simulink model "HTdieukhiennhietdophong"  (R2017b)
settings: Solver=VariableStepAuto  StartTime=0.0  StopTime=200  RelTol=1e-3
libraries: simulink x2
settings Model: Creator=chemi  LastModifiedBy=chemi

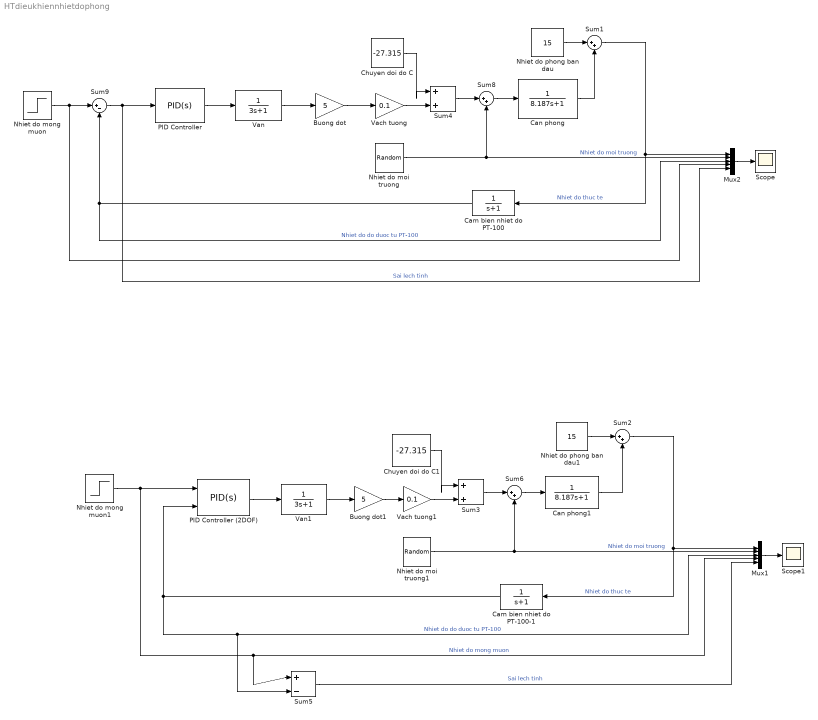
== system HTdieukhiennhietdophong ==
  Buong dot : Gain  Gain=5
  Buong dot1 : Gain  Gain=5
  Cam bien nhiet do PT-100 : TransferFcn  Denominator=[1 1]
  Cam bien nhiet do PT-100-1 : TransferFcn  Denominator=[1 1]
  Can phong : TransferFcn  Denominator=[8.187 1]
  Can phong1 : TransferFcn  Denominator=[8.187 1]
  Chuyen doi do C : Constant  Value=-27.315
  Chuyen doi do C1 : Constant  Value=-27.315
  Mux1 : Mux  Inputs=5
  Mux2 : Mux  Inputs=5
  Nhiet do mong muon : Step  Time=0  After=25  SampleTime=0
  Nhiet do mong muon1 : Step  Time=0  After=25  SampleTime=0
  Nhiet do moi truong : RandomNumber  Mean=13  Seed=5  SampleTime=7
  Nhiet do moi truong1 : RandomNumber  Mean=13  Seed=5  SampleTime=7
  Nhiet do phong ban dau : Constant  Value=15
  Nhiet do phong ban dau1 : Constant  Value=15
  PID Controller : simulink/Continuous/PID Controller  Controller=PID  TimeDomain=Continuous-time  SampleTime=-1  IntegratorMethod=Forward Euler  FilterMethod=Forward Euler  Form=Parallel  UseFilter=on  ControllerParametersSource=internal  P=10.9392711436423  I=0.847145047333373  D=35.2294426179571  N=64.8599960796025  InitialConditionSource=internal  InitialConditionForIntegrator=0  InitialConditionForFilter=0  ExternalReset=none  LimitOutput=on  UpperSaturationLimit=100  LowerSaturationLimit=0  LinearizeAsGain=on  AntiWindupMode=none  Kb=1  TrackingMode=off  Kt=1  PParamMin=[]  PParamMax=[]  IParamMin=[]  IParamMax=[]  DParamMin=[]  DParamMax=[]  NParamMin=[]  NParamMax=[]  KbParamMin=[]  KbParamMax=[]  KtParamMin=[]  KtParamMax=[]  POutMin=[]  POutMax=[]  IOutMin=[]  IOutMax=[]  DOutMin=[]  DOutMax=[]  NOutMin=[]  NOutMax=[]  KbOutMin=[]  KbOutMax=[]  KtOutMin=[]  KtOutMax=[]  IntegratorOutMin=[]  IntegratorOutMax=[]  FilterOutMin=[]  FilterOutMax=[]  SumOutMin=[]  SumOutMax=[]  SumI1OutMin=[]  SumI1OutMax=[]  SumI2OutMin=[]  SumI2OutMax=[]  SumI3OutMin=[]  SumI3OutMax=[]  SumDOutMin=[]  SumDOutMax=[]  SaturationOutMin=[]  SaturationOutMax=[]  IntegratorContinuousStateAttributes=''  IntegratorStateMustResolveToSignalObject=off  IntegratorRTWStateStorageClass=Auto  FilterContinuousStateAttributes=''  FilterStateMustResolveToSignalObject=off  FilterRTWStateStorageClass=Auto  DifferentiatorICPrevScaledInput=0  DifferentiatorOutMin=[]  DifferentiatorOutMax=[]  InitialConditionSetting=State (most efficient)  FilterDiffOutCoefMin=[]  FilterDiffOutCoefMax=[]  SumDenOutMin=[]  SumDenOutMax=[]  SumNumOutMin=[]  SumNumOutMax=[]  ReciprocalOutMin=[]  ReciprocalOutMax=[]  DivideOutMin=[]  DivideOutMax=[]  TunerSelectOption=Transfer Function Based (PID Tuner App)
  PID Controller (2DOF) : simulink/Continuous/PID Controller (2DOF)  Controller=PID  TimeDomain=Continuous-time  SampleTime=-1  IntegratorMethod=Forward Euler  FilterMethod=Forward Euler  Form=Parallel  UseFilter=on  ControllerParametersSource=internal  P=30.7497062437727  I=4.09275369007952  D=55.8944403669847  N=9.43538808450386  b=0.544641384647558  c=0.0108926766550365  InitialConditionSource=internal  InitialConditionForIntegrator=0  InitialConditionForFilter=0  ExternalReset=none  LimitOutput=on  UpperSaturationLimit=100  LowerSaturationLimit=0  LinearizeAsGain=on  AntiWindupMode=none  Kb=1  TrackingMode=off  Kt=1  PParamMin=[]  PParamMax=[]  IParamMin=[]  IParamMax=[]  DParamMin=[]  DParamMax=[]  NParamMin=[]  NParamMax=[]  bParamMin=[]  bParamMax=[]  cParamMin=[]  cParamMax=[]  KbParamMin=[]  KbParamMax=[]  KtParamMin=[]  KtParamMax=[]  POutMin=[]  POutMax=[]  IOutMin=[]  IOutMax=[]  DOutMin=[]  DOutMax=[]  NOutMin=[]  NOutMax=[]  bOutMin=[]  bOutMax=[]  cOutMin=[]  cOutMax=[]  KbOutMin=[]  KbOutMax=[]  KtOutMin=[]  KtOutMax=[]  IntegratorOutMin=[]  IntegratorOutMax=[]  FilterOutMin=[]  FilterOutMax=[]  SumOutMin=[]  SumOutMax=[]  Sum1OutMin=[]  Sum1OutMax=[]  Sum2OutMin=[]  Sum2OutMax=[]  Sum3OutMin=[]  Sum3OutMax=[]  SumI1OutMin=[]  SumI1OutMax=[]  SumI2OutMin=[]  SumI2OutMax=[]  SumI3OutMin=[]  SumI3OutMax=[]  SumDOutMin=[]  SumDOutMax=[]  SaturationOutMin=[]  SaturationOutMax=[]  IntegratorContinuousStateAttributes=''  IntegratorStateMustResolveToSignalObject=off  IntegratorRTWStateStorageClass=Auto  FilterContinuousStateAttributes=''  FilterStateMustResolveToSignalObject=off  FilterRTWStateStorageClass=Auto  DifferentiatorICPrevScaledInput=0  DifferentiatorOutMin=[]  DifferentiatorOutMax=[]  InitialConditionSetting=State (most efficient)  FilterDiffOutCoefMin=[]  FilterDiffOutCoefMax=[]  SumDenOutMin=[]  SumDenOutMax=[]  SumNumOutMin=[]  SumNumOutMax=[]  ReciprocalOutMin=[]  ReciprocalOutMax=[]  DivideOutMin=[]  DivideOutMax=[]  TunerSelectOption=Transfer Function Based (PID Tuner App)
  Scope : Scope
  Scope1 : Scope
  Sum{1..4,6,8} (6 alike) : Sum  Inputs=|++
  Sum5 : Sum  Inputs=|+-
  Sum9 : Sum  Inputs=|+-
  Vach tuong : Gain  Gain=0.1
  Vach tuong1 : Gain  Gain=0.1
  Van : TransferFcn  Denominator=[3 1]
  Van1 : TransferFcn  Denominator=[3 1]
  wires:
  Nhiet do mong muon1/1 -> PID Controller (2DOF)/1, Mux1/4, Sum5/1  "Nhiet do mong muon"
  Sum2/1 -> Cam bien nhiet do PT-100-1/1, Mux1/1  "Nhiet do thuc te"
  Vach tuong1/1 -> Sum3/2
  Sum6/1 -> Can phong1/1
  Sum3/1 -> Sum6/1
  Can phong1/1 -> Sum2/2
  Nhiet do phong ban dau1/1 -> Sum2/1
  Nhiet do moi truong1/1 -> Mux1/2, Sum6/2  "Nhiet do moi truong"
  Chuyen doi do C1/1 -> Sum3/1
  Mux1/1 -> Scope1/1
  Cam bien nhiet do PT-100-1/1 -> PID Controller (2DOF)/2, Sum5/2, Mux1/3  "Nhiet do do duoc tu PT-100"
  Sum5/1 -> Mux1/5  "Sai lech tinh"
  Mux2/1 -> Scope/1
  Cam bien nhiet do PT-100/1 -> Sum9/2, Mux2/3  "Nhiet do do duoc tu PT-100"
  Nhiet do moi truong/1 -> Mux2/2, Sum8/2  "Nhiet do moi truong"
  Nhiet do phong ban dau/1 -> Sum1/1
  Buong dot/1 -> Vach tuong/1
  Sum1/1 -> Cam bien nhiet do PT-100/1, Mux2/1  "Nhiet do thuc te"
  PID Controller/1 -> Van/1
  Sum9/1 -> Mux2/5, PID Controller/1  "Sai lech tinh"
  Can phong/1 -> Sum1/2
  Sum8/1 -> Can phong/1
  Van/1 -> Buong dot/1
  Nhiet do mong muon/1 -> Sum9/1, Mux2/4
  Sum4/1 -> Sum8/1
  Chuyen doi do C/1 -> Sum4/1
  Vach tuong/1 -> Sum4/2
  Buong dot1/1 -> Vach tuong1/1
  Van1/1 -> Buong dot1/1
  PID Controller (2DOF)/1 -> Van1/1
